simulink model "simulink_test_fcn_timeSeriesVehicleTrajectory"  (R2019b)
settings: Solver=FixedStepAuto  StartTime=0.0  StopTime=45  FixedStep=0.01  RelTol=1e-4  EnableMultiTasking=on
settings Model: Creator=cbeal  LastModifiedBy=prasa
settings SolverCC: ZeroCrossAlgorithm=Adaptive
settings DataIOCC: SaveFormat=Array  SignalLoggingSaveFormat=ModelDataLogs  ReturnWorkspaceOutputs=off
settings OptimizationCC: ExpressionDepthLimit=2147483647  LifeSpan=inf
settings DebuggingCC: UnderspecifiedInitializationDetection=Classic  MergeDetectMultiDrivingBlocksExec=none  SolverPrmCheckMsg=warning  FcnCallInpInsideContextMsg=warning  StateNameClashWarn=warning  SFUnexpectedBacktrackingDiag=warning  SFNoUnconditionalDefaultTransitionDiag=warning  SFExecutionAtInitializationDiag=none  ArithmeticOperatorsInVariantConditions=warning
settings HardwareCC: ProdBitPerPointer=32  ProdBitPerSizeT=32  ProdBitPerPtrDiffT=32  ProdLargestAtomicFloat=None  ProdIntDivRoundTo=Undefined  ProdEndianess=Unspecified  ProdWordSize=32  ProdHWDeviceType=32-bit Generic
settings ModelReferenceCC: PropagateSignalLabelsOutOfModel=off
settings SFSimCC: SimUseLocalCustomCode=off  CustomCodeUndefinedFunction=UseInterfaceOnly
settings RTWCC: RTWUseLocalCustomCode=off
settings CodeAppCC: StateflowObjectComments=on
settings GRTTargetCC: TargetLangStandard=C89/C90 (ANSI)  GeneratePreprocessorConditionals=Disable all
settings ConfigComp: CovMetricSettings=dw  CovHtmlReporting=on  CovSaveCumulativeToWorkspaceVar=on  CovSaveSingleToWorkspaceVar=on  CovExternalEMLEnable=off

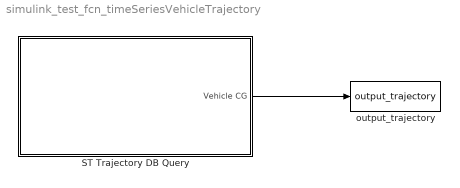
== system simulink_test_fcn_timeSeriesVehicleTrajectory ==
  ST Trajectory DB Query : Subsystem
  output_trajectory : ToWorkspace  VariableName=output_trajectory  SampleTime=-1
      settings: Save2DSignal=2-D array (concatenate along first dimension)
  wires:
  ST Trajectory DB Query/1(Vehicle CG) -> output_trajectory/1

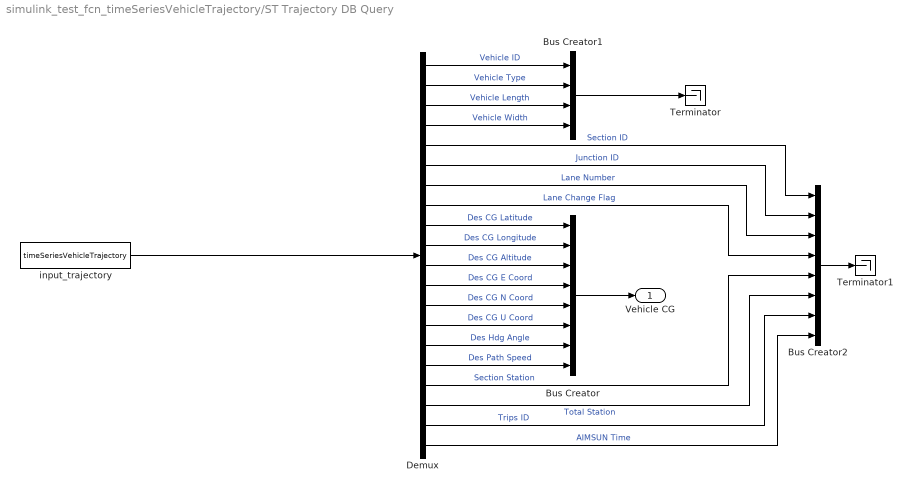
== system simulink_test_fcn_timeSeriesVehicleTrajectory/ST Trajectory DB Query ==
  Bus Creator : BusCreator  Inputs=8
  Bus Creator1 : BusCreator  Inputs=4
  Bus Creator2 : BusCreator  Inputs=8
  Demux : Demux  Outputs=20
  Terminator : Terminator
  Terminator1 : Terminator
  input_trajectory : FromWorkspace  VariableName=timeSeriesVehicleTrajectory  OutputAfterFinalValue=Holding final value
  Vehicle CG : Outport
  wires:
  Demux/1 -> Bus Creator1/1  "Vehicle ID"
  Demux/2 -> Bus Creator1/2  "Vehicle Type"
  Demux/3 -> Bus Creator1/3  "Vehicle Length"
  Demux/4 -> Bus Creator1/4  "Vehicle Width"
  Demux/5 -> Bus Creator2/1  "Section ID"
  Demux/6 -> Bus Creator2/2  "Junction ID"
  Demux/7 -> Bus Creator2/3  "Lane Number"
  Demux/8 -> Bus Creator2/4  "Lane Change Flag"
  Demux/9 -> Bus Creator/1  "Des CG Latitude"
  Demux/10 -> Bus Creator/2  "Des CG Longitude"
  Demux/11 -> Bus Creator/3  "Des CG Altitude"
  Demux/12 -> Bus Creator/4  "Des CG E Coord"
  Demux/13 -> Bus Creator/5  "Des CG N Coord"
  Demux/14 -> Bus Creator/6  "Des CG U Coord"
  Demux/15 -> Bus Creator/7  "Des Hdg Angle"
  Demux/16 -> Bus Creator/8  "Des Path Speed"
  Demux/17 -> Bus Creator2/5  "Section Station"
  Demux/18 -> Bus Creator2/6  "Total Station"
  Demux/20 -> Bus Creator2/8  "AIMSUN Time"
  Demux/19 -> Bus Creator2/7  "Trips ID"
  Bus Creator1/1 -> Terminator/1
  Bus Creator/1 -> Vehicle CG/1
  Bus Creator2/1 -> Terminator1/1
  input_trajectory/1 -> Demux/1
